simulink model "ex3sim"  (R2015a)
settings: Solver=ode45  StartTime=0.0  StopTime=1  RelTol=1e-3
undefined symbols (not defined in the file): Ts
settings Model: Creator=BPeixoto  LastModifiedBy=BPeixoto

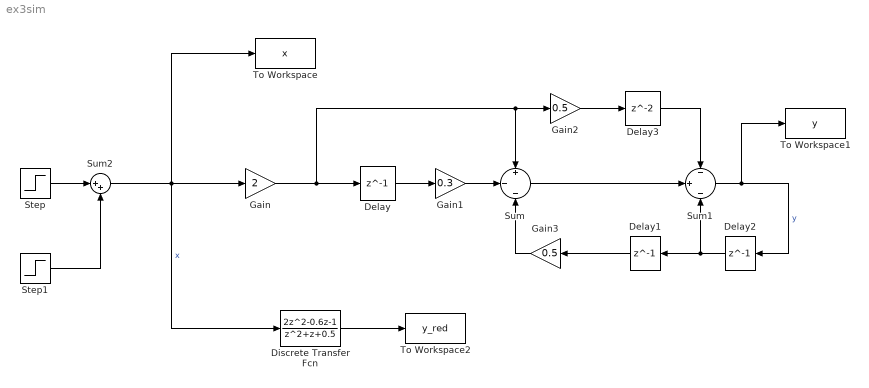
== system ex3sim ==
  Delay : Delay  DelayLength=1  InitialCondition=0  SampleTime=Ts
  Delay1 : Delay  DelayLength=1  InitialCondition=0  SampleTime=Ts
  Delay2 : Delay  DelayLength=1  InitialCondition=0  SampleTime=Ts
  Delay3 : Delay  InitialCondition=0  SampleTime=Ts
  Discrete Transfer Fcn : DiscreteTransferFcn  Numerator=[2, -0.6, -1]  Denominator=[1, 1, 0.5]  SampleTime=Ts
  Gain : Gain  Gain=2
  Gain1 : Gain  Gain=0.3
  Gain2 : Gain  Gain=0.5
  Gain3 : Gain  Gain=0.5
  Step : Step  Time=Ts  SampleTime=0
  Step1 : Step  Time=3*Ts  After=-1  SampleTime=0
  Sum : Sum  Inputs=+|-|-
  Sum1 : Sum  Inputs=-|+|-
  Sum2 : Sum  Inputs=|++
  To Workspace : ToWorkspace  VariableName=x  SaveFormat=Structure With Time  SampleTime=-1
  To Workspace1 : ToWorkspace  VariableName=y  SaveFormat=Structure With Time  SampleTime=-1
  To Workspace2 : ToWorkspace  VariableName=y_red  SaveFormat=Structure With Time  SampleTime=-1
  wires:
  Gain/1 -> Delay/1, Sum/1, Gain2/1
  Delay/1 -> Gain1/1
  Gain1/1 -> Sum/2
  Gain3/1 -> Sum/3
  Delay1/1 -> Gain3/1
  Delay2/1 -> Sum1/3, Delay1/1
  Sum/1 -> Sum1/2
  Gain2/1 -> Delay3/1
  Delay3/1 -> Sum1/1
  Sum1/1 -> To Workspace1/1, Delay2/1  "y"
  Sum2/1 -> Gain/1, To Workspace/1, Discrete Transfer Fcn/1  "x"
  Step/1 -> Sum2/1
  Step1/1 -> Sum2/2
  Discrete Transfer Fcn/1 -> To Workspace2/1
